simulink model "ADRC"  (R2018b)
settings: configuration reference "Configuration" (kept outside this file)
undefined symbols (not defined in the file): DiscIntNeverNeededParam
libraries: adrc_lib x1
settings Model: Creator=zouji  LastModifiedBy=zouji
settings ConfigSetRef: SourceLocation=Base Workspace

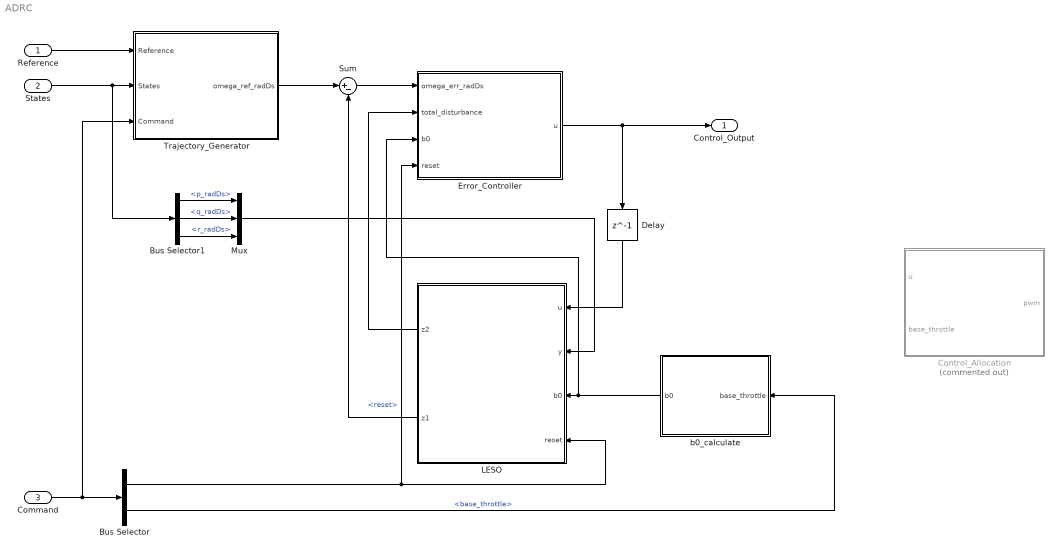
== system ADRC ==
  Reference : Inport  OutDataTypeStr=Bus: Reference
  States : Inport  Port=2  OutDataTypeStr=Bus: States
  Command : Inport  Port=3  OutDataTypeStr=Bus: Command
  Bus Selector : BusSelector  OutputSignals=reset,base_throttle
  Bus Selector1 : BusSelector  OutputSignals=p_radDs,q_radDs,r_radDs
  Control_Allocation : Subsystem  Commented=on
  Delay : Delay  DelayLength=1
  Error_Controller : Subsystem
  LESO : Subsystem  mask{beta1=0, beta2=0}
  Mux : Mux  Inputs=3
  Sum : Sum  Inputs=|+-
  Trajectory_Generator : Subsystem  mask{r1=0, h1=0}
  b0_calculate : Subsystem  mask{k=0, cT=0, l=0, p=0, Ixx=0, Iyy=0, Izz=0}
      mask prompts: l "arm length"
  Control_Output : Outport  OutDataTypeStr=Bus: Control_Output
  wires:
  Reference/1 -> Trajectory_Generator/1(Reference)
  States/1 -> Bus Selector1/1, Trajectory_Generator/2(States)
  Bus Selector1/1 -> Mux/1  "<p_radDs>"
  Bus Selector1/2 -> Mux/2  "<q_radDs>"
  Bus Selector1/3 -> Mux/3  "<r_radDs>"
  Trajectory_Generator/1(omega_ref_radDs) -> Sum/1
  Error_Controller/1(u) -> Control_Output/1, Delay/1
  Sum/1 -> Error_Controller/1(omega_err_radDs)
  LESO/1(z2) -> Error_Controller/2(total_disturbance)
  LESO/2(z1) -> Sum/2
  Delay/1 -> LESO/1(u)
  Mux/1 -> LESO/2(y)
  Command/1 -> Trajectory_Generator/3(Command), Bus Selector/1
  Bus Selector/1 -> Error_Controller/4(reset), LESO/4(reset)  "<reset>"
  Bus Selector/2 -> b0_calculate/1(base_throttle)  "<base_throttle>"
  b0_calculate/1(b0) -> Error_Controller/3(b0), LESO/3(b0)

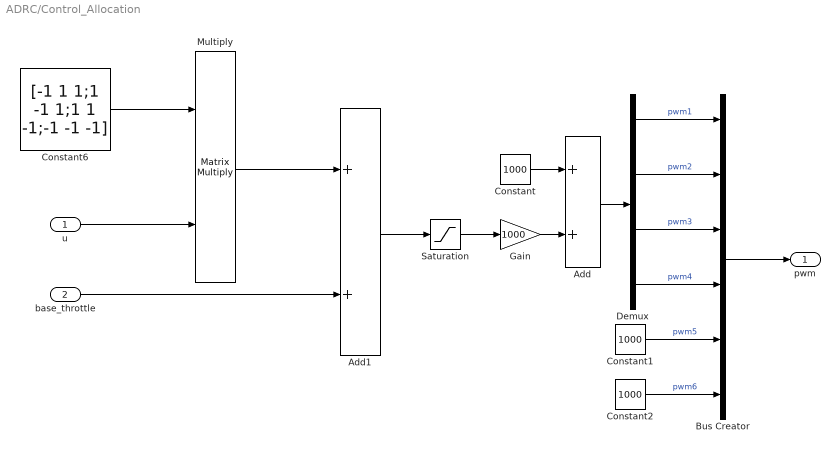
== system ADRC/Control_Allocation ==
  u : Inport
  base_throttle : Inport  Port=2
  Add : Sum
  Add1 : Sum
  Bus Creator : BusCreator  Inputs=6
  Constant : Constant  Value=1000  OutDataTypeStr=int16
  Constant1 : Constant  Value=1000  OutDataTypeStr=int16
  Constant2 : Constant  Value=1000  OutDataTypeStr=int16
  Constant6 : Constant  Value=[-1 1 1;1 -1 1;1 1 -1;-1 -1 -1]  OutDataTypeStr=single
  Demux : Demux
  Gain : Gain  Gain=1000  OutDataTypeStr=int16
  Multiply : Product  Multiplication=Matrix(*)  OutDataTypeStr=Inherit: Same as first input
  Saturation : Saturate  UpperLimit=1  LowerLimit=0
  pwm : Outport
  wires:
  Demux/1 -> Bus Creator/1  "pwm1"
  Constant/1 -> Add/1
  Add1/1 -> Saturation/1
  Demux/3 -> Bus Creator/3  "pwm3"
  Bus Creator/1 -> pwm/1
  Constant2/1 -> Bus Creator/6  "pwm6"
  Gain/1 -> Add/2
  Add/1 -> Demux/1
  Demux/4 -> Bus Creator/4  "pwm4"
  u/1 -> Multiply/2
  Demux/2 -> Bus Creator/2  "pwm2"
  Constant6/1 -> Multiply/1
  Multiply/1 -> Add1/1
  Constant1/1 -> Bus Creator/5  "pwm5"
  base_throttle/1 -> Add1/2
  Saturation/1 -> Gain/1

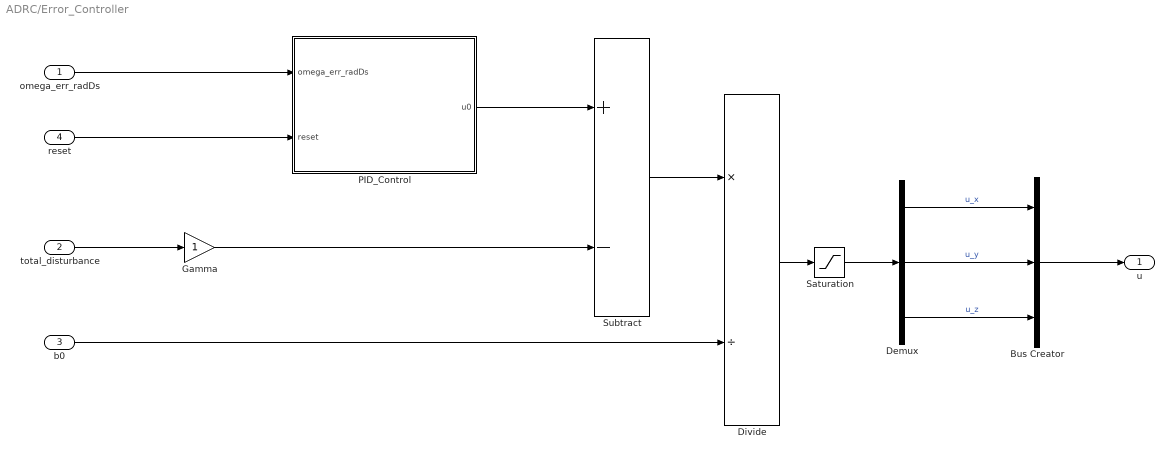
== system ADRC/Error_Controller ==
  omega_err_radDs : Inport
  total_disturbance : Inport  Port=2
  b0 : Inport  Port=3
  reset : Inport  Port=4
  Bus Creator : BusCreator  Inputs=3
  Demux : Demux  Outputs=3
  Divide : Product  Inputs=*/  OutDataTypeStr=Inherit: Same as first input
  Gamma : Gain
  PID_Control : Subsystem
  Saturation : Saturate
  Subtract : Sum  Inputs=+-
  u : Outport
  wires:
  omega_err_radDs/1 -> PID_Control/1(omega_err_radDs)
  total_disturbance/1 -> Gamma/1
  Divide/1 -> Saturation/1
  reset/1 -> PID_Control/2(reset)
  Gamma/1 -> Subtract/2
  PID_Control/1(u0) -> Subtract/1
  Subtract/1 -> Divide/1
  b0/1 -> Divide/2
  Saturation/1 -> Demux/1
  Demux/1 -> Bus Creator/1  "u_x"
  Demux/2 -> Bus Creator/2  "u_y"
  Demux/3 -> Bus Creator/3  "u_z"
  Bus Creator/1 -> u/1

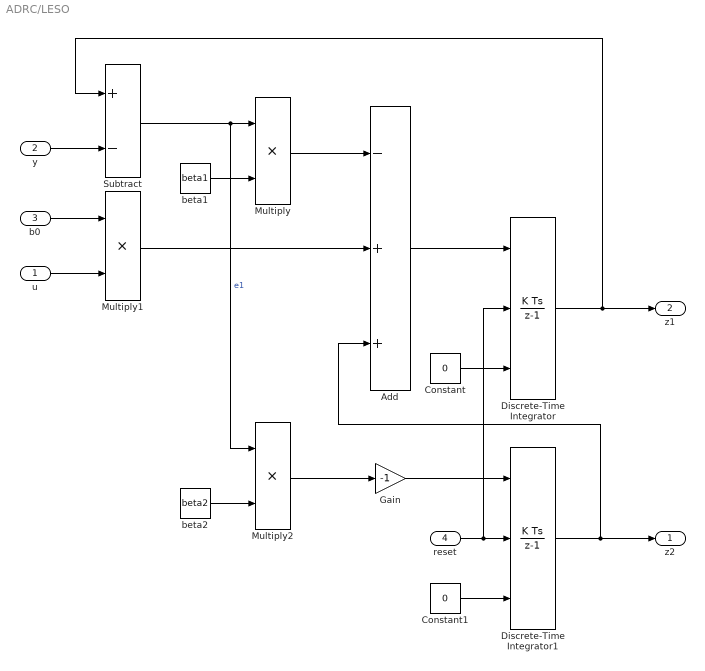
== system ADRC/LESO ==
  u : Inport
  y : Inport  Port=2
  b0 : Inport  Port=3
  reset : Inport  Port=4
  Add : Sum  Inputs=-++
  Constant : Constant  Value=0  OutDataTypeStr=single
  Constant1 : Constant  Value=0  OutDataTypeStr=single
  Discrete-Time Integrator : DiscreteIntegrator  ExternalReset=level  InitialConditionSource=external  SampleTime=-1  ICPrevOutput=DiscIntNeverNeededParam  ICPrevScaledInput=DiscIntNeverNeededParam
  Discrete-Time Integrator1 : DiscreteIntegrator  ExternalReset=level  InitialConditionSource=external  SampleTime=-1  ICPrevOutput=DiscIntNeverNeededParam  ICPrevScaledInput=DiscIntNeverNeededParam
  Gain : Gain  Gain=-1  OutDataTypeStr=Inherit: Same as input
  Multiply : Product  OutDataTypeStr=Inherit: Same as first input
  Multiply1 : Product  OutDataTypeStr=Inherit: Same as first input
  Multiply2 : Product  OutDataTypeStr=Inherit: Same as first input
  Subtract : Sum  Inputs=+-
  beta1 : Constant  Value=beta1  OutDataTypeStr=single
  beta2 : Constant  Value=beta2  OutDataTypeStr=single
  z2 : Outport
  z1 : Outport  Port=2
  wires:
  Discrete-Time Integrator/1 -> Subtract/1, z1/1
  Discrete-Time Integrator1/1 -> Add/3, z2/1
  y/1 -> Subtract/2
  Subtract/1 -> Multiply/1, Multiply2/1  "e1"
  Add/1 -> Discrete-Time Integrator/1
  Multiply/1 -> Add/1
  beta1/1 -> Multiply/2
  Multiply1/1 -> Add/2
  b0/1 -> Multiply1/1
  u/1 -> Multiply1/2
  Multiply2/1 -> Gain/1
  beta2/1 -> Multiply2/2
  Gain/1 -> Discrete-Time Integrator1/1
  Constant/1 -> Discrete-Time Integrator/3
  Constant1/1 -> Discrete-Time Integrator1/3
  reset/1 -> Discrete-Time Integrator1/2, Discrete-Time Integrator/2

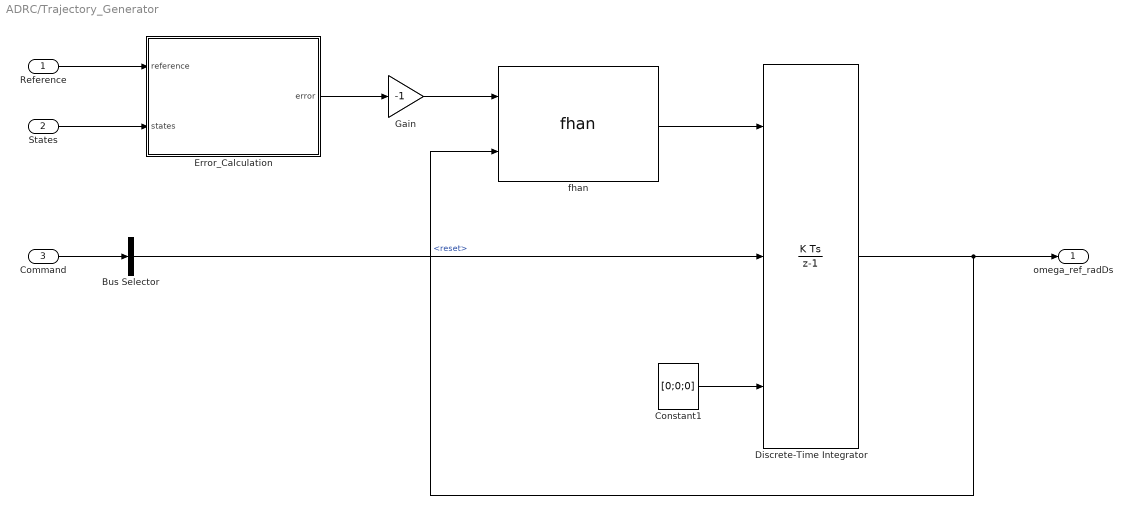
== system ADRC/Trajectory_Generator ==
  Reference : Inport
  States : Inport  Port=2
  Command : Inport  Port=3
  Bus Selector : BusSelector  OutputSignals=reset
  Constant1 : Constant  Value=[0;0;0]  OutDataTypeStr=single
  Discrete-Time Integrator : DiscreteIntegrator  ExternalReset=level  InitialConditionSource=external  SampleTime=-1  ICPrevOutput=DiscIntNeverNeededParam  ICPrevScaledInput=DiscIntNeverNeededParam
  Error_Calculation : Subsystem
  Gain : Gain  Gain=-1  OutDataTypeStr=Inherit: Same as input
  fhan : adrc_lib/fhan  r0=r1  h0=h1
  omega_ref_radDs : Outport
  wires:
  Reference/1 -> Error_Calculation/1(reference)
  States/1 -> Error_Calculation/2(states)
  Error_Calculation/1(error) -> Gain/1
  Gain/1 -> fhan/1
  fhan/1 -> Discrete-Time Integrator/1
  Command/1 -> Bus Selector/1
  Bus Selector/1 -> Discrete-Time Integrator/2  "<reset>"
  Constant1/1 -> Discrete-Time Integrator/3
  Discrete-Time Integrator/1 -> omega_ref_radDs/1, fhan/2

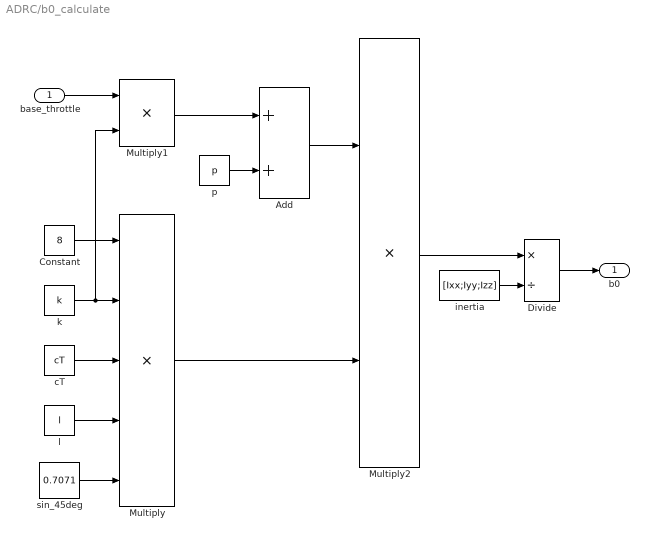
== system ADRC/b0_calculate ==
  base_throttle : Inport
  Add : Sum
  Constant : Constant  Value=8  OutDataTypeStr=single
  Divide : Product  Inputs=*/  OutDataTypeStr=Inherit: Same as first input
  Multiply : Product  Inputs=5  OutDataTypeStr=Inherit: Same as first input
  Multiply1 : Product  OutDataTypeStr=Inherit: Same as first input
  Multiply2 : Product  OutDataTypeStr=Inherit: Same as first input
  cT : Constant  Value=cT  OutDataTypeStr=single
  inertia : Constant  Value=[Ixx;Iyy;Izz]  OutDataTypeStr=single
  k : Constant  Value=k  OutDataTypeStr=single
  l : Constant  Value=l  OutDataTypeStr=single
  p : Constant  Value=p  OutDataTypeStr=single
  sin_45deg : Constant  Value=0.7071
  b0 : Outport
  wires:
  Constant/1 -> Multiply/1
  k/1 -> Multiply/2, Multiply1/2
  cT/1 -> Multiply/3
  l/1 -> Multiply/4
  sin_45deg/1 -> Multiply/5
  base_throttle/1 -> Multiply1/1
  Multiply1/1 -> Add/1
  p/1 -> Add/2
  Add/1 -> Multiply2/1
  Multiply/1 -> Multiply2/2
  Multiply2/1 -> Divide/1
  inertia/1 -> Divide/2
  Divide/1 -> b0/1

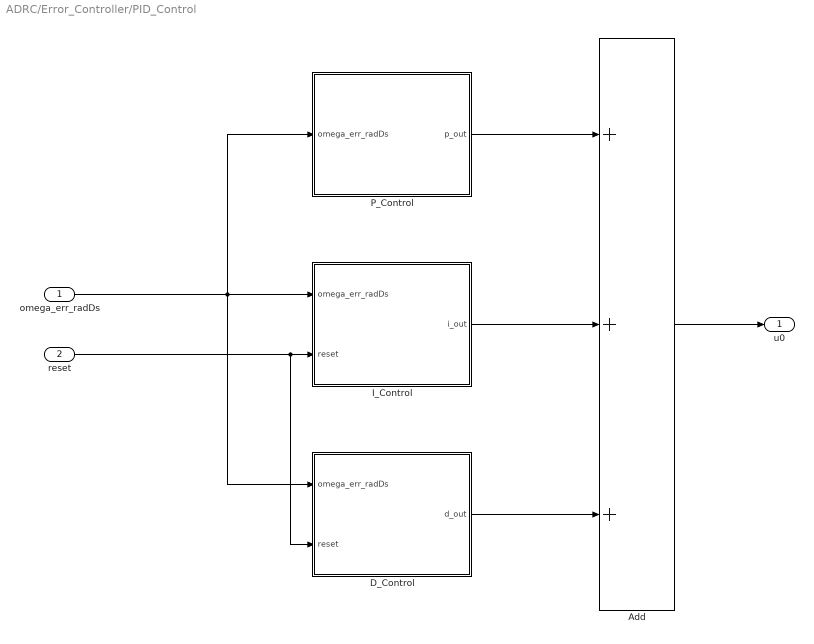
== system ADRC/Error_Controller/PID_Control ==
  omega_err_radDs : Inport
  reset : Inport  Port=2
  Add : Sum  Inputs=+++
  D_Control : Subsystem  mask{r_kd=1, p_kd=1, q_kd=1, max_d=0.2, min_d=-0.2}
  I_Control : Subsystem  mask{r_ki=1, p_ki=1, q_ki=1, max_i=0.2, min_i=-0.2}
  P_Control : Subsystem  mask{r_kp=1, p_kp=1, q_kp=1}
  u0 : Outport
  wires:
  omega_err_radDs/1 -> P_Control/1(omega_err_radDs), I_Control/1(omega_err_radDs), D_Control/1(omega_err_radDs)
  reset/1 -> I_Control/2(reset), D_Control/2(reset)
  P_Control/1(p_out) -> Add/1
  I_Control/1(i_out) -> Add/2
  D_Control/1(d_out) -> Add/3
  Add/1 -> u0/1

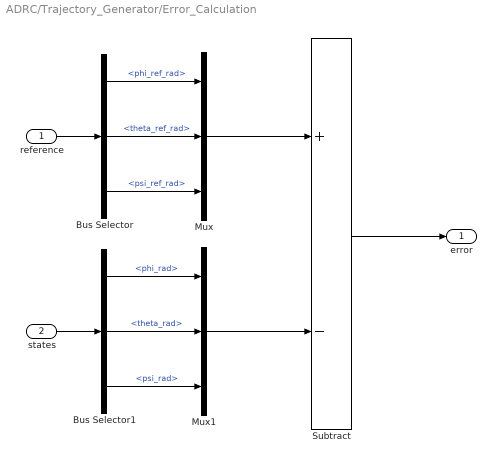
== system ADRC/Trajectory_Generator/Error_Calculation ==
  reference : Inport
  states : Inport  Port=2
  Bus Selector : BusSelector  OutputSignals=phi_ref_rad,theta_ref_rad,psi_ref_rad
  Bus Selector1 : BusSelector  OutputSignals=phi_rad,theta_rad,psi_rad
  Mux : Mux  Inputs=3
  Mux1 : Mux  Inputs=3
  Subtract : Sum  Inputs=+-
  error : Outport
  wires:
  reference/1 -> Bus Selector/1
  Bus Selector/1 -> Mux/1  "<phi_ref_rad>"
  Bus Selector/2 -> Mux/2  "<theta_ref_rad>"
  Bus Selector/3 -> Mux/3  "<psi_ref_rad>"
  Bus Selector1/2 -> Mux1/2  "<theta_rad>"
  Bus Selector1/3 -> Mux1/3  "<psi_rad>"
  Bus Selector1/1 -> Mux1/1  "<phi_rad>"
  states/1 -> Bus Selector1/1
  Mux/1 -> Subtract/1
  Mux1/1 -> Subtract/2
  Subtract/1 -> error/1

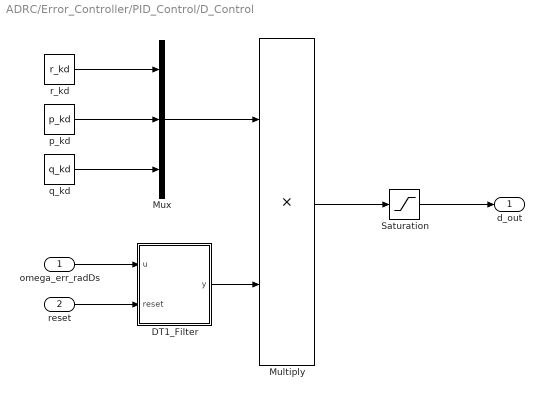
== system ADRC/Error_Controller/PID_Control/D_Control ==
  omega_err_radDs : Inport
  reset : Inport  Port=2
  DT1_Filter : Subsystem  mask{T_filter=0.1}
      mask prompts: T_filter "Time constant [s]"
      mask Display: fprintf('T = %.3f', T_filter)
  Multiply : Product  OutDataTypeStr=Inherit: Same as first input
  Mux : Mux  Inputs=3
  Saturation : Saturate  UpperLimit=max_d  LowerLimit=min_d
  p_kd : Constant  Value=p_kd  OutDataTypeStr=single
  q_kd : Constant  Value=q_kd  OutDataTypeStr=single
  r_kd : Constant  Value=r_kd  OutDataTypeStr=single
  d_out : Outport
  wires:
  omega_err_radDs/1 -> DT1_Filter/1(u)
  p_kd/1 -> Mux/2
  Mux/1 -> Multiply/1
  r_kd/1 -> Mux/1
  Multiply/1 -> Saturation/1
  q_kd/1 -> Mux/3
  DT1_Filter/1(y) -> Multiply/2
  Saturation/1 -> d_out/1
  reset/1 -> DT1_Filter/2(reset)

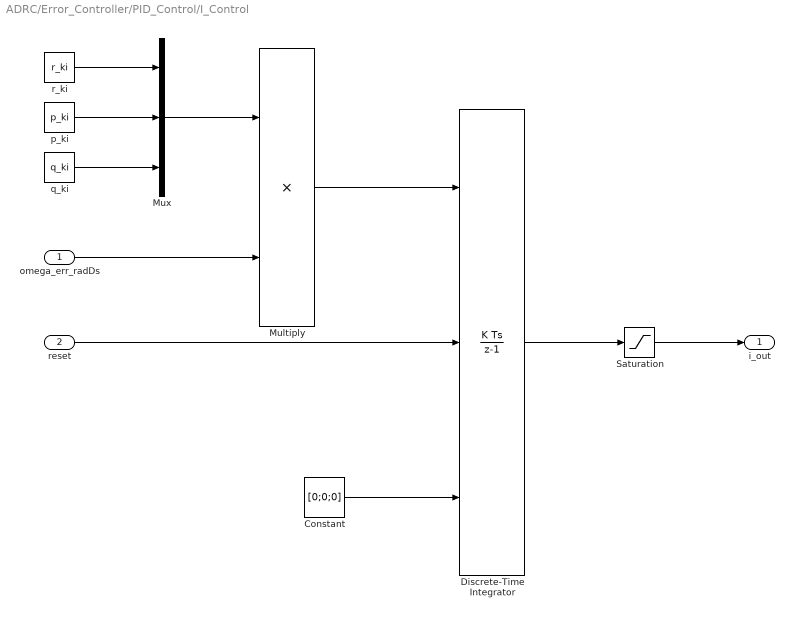
== system ADRC/Error_Controller/PID_Control/I_Control ==
  omega_err_radDs : Inport
  reset : Inport  Port=2
  Constant : Constant  Value=[0;0;0]  OutDataTypeStr=single
  Discrete-Time Integrator : DiscreteIntegrator  ExternalReset=level  InitialConditionSource=external  SampleTime=-1  ICPrevOutput=DiscIntNeverNeededParam  ICPrevScaledInput=DiscIntNeverNeededParam
  Multiply : Product  OutDataTypeStr=Inherit: Same as first input
  Mux : Mux  Inputs=3
  Saturation : Saturate  UpperLimit=max_i  LowerLimit=min_i
  p_ki : Constant  Value=p_ki  OutDataTypeStr=single
  q_ki : Constant  Value=q_ki  OutDataTypeStr=single
  r_ki : Constant  Value=r_ki  OutDataTypeStr=single
  i_out : Outport
  wires:
  omega_err_radDs/1 -> Multiply/2
  p_ki/1 -> Mux/2
  Mux/1 -> Multiply/1
  r_ki/1 -> Mux/1
  q_ki/1 -> Mux/3
  Multiply/1 -> Discrete-Time Integrator/1
  reset/1 -> Discrete-Time Integrator/2
  Constant/1 -> Discrete-Time Integrator/3
  Discrete-Time Integrator/1 -> Saturation/1
  Saturation/1 -> i_out/1

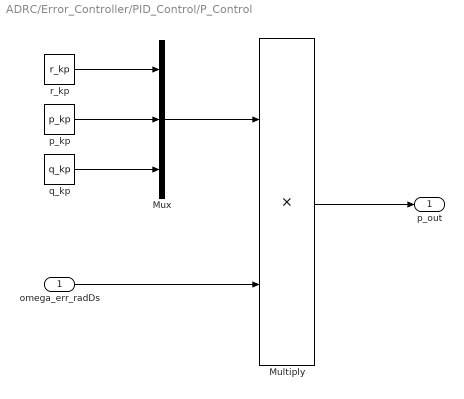
== system ADRC/Error_Controller/PID_Control/P_Control ==
  omega_err_radDs : Inport
  Multiply : Product  OutDataTypeStr=Inherit: Same as first input
  Mux : Mux  Inputs=3
  p_kp : Constant  Value=p_kp  OutDataTypeStr=single
  q_kp : Constant  Value=q_kp  OutDataTypeStr=single
  r_kp : Constant  Value=r_kp  OutDataTypeStr=single
  p_out : Outport
  wires:
  omega_err_radDs/1 -> Multiply/2
  p_kp/1 -> Mux/2
  Mux/1 -> Multiply/1
  r_kp/1 -> Mux/1
  Multiply/1 -> p_out/1
  q_kp/1 -> Mux/3

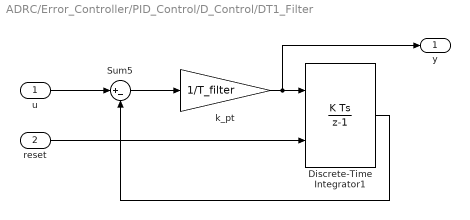
== system ADRC/Error_Controller/PID_Control/D_Control/DT1_Filter ==
  u : Inport
  reset : Inport  Port=2
  Discrete-Time Integrator1 : DiscreteIntegrator  ExternalReset=level  SampleTime=-1  ICPrevOutput=DiscIntNeverNeededParam  ICPrevScaledInput=DiscIntNeverNeededParam
  Sum5 : Sum  Inputs=|+-
  k_pt : Gain  Gain=1/T_filter  OutDataTypeStr=Inherit: Same as input
  y : Outport
  wires:
  u/1 -> Sum5/1
  Sum5/1 -> k_pt/1
  Discrete-Time Integrator1/1 -> Sum5/2
  k_pt/1 -> Discrete-Time Integrator1/1, y/1
  reset/1 -> Discrete-Time Integrator1/2
